simulink model "MatlabCode"  (R2017b)
settings: Solver=FixedStepDiscrete  StartTime=0.0  StopTime=inf  RelTol=1e-3
PreLoadFcn:
  | waijung.modelPreload; % Required for working with Waijung Blockset. Do not remove.
undefined symbols (not defined in the file): HSEOSC, Link, LQFP100, ST, STM32F407VG
libraries: stm32f4_io_lib x6, stm32f4_adc_lib x1, stm32f4_device_config_lib x1
(part 2 of 2)

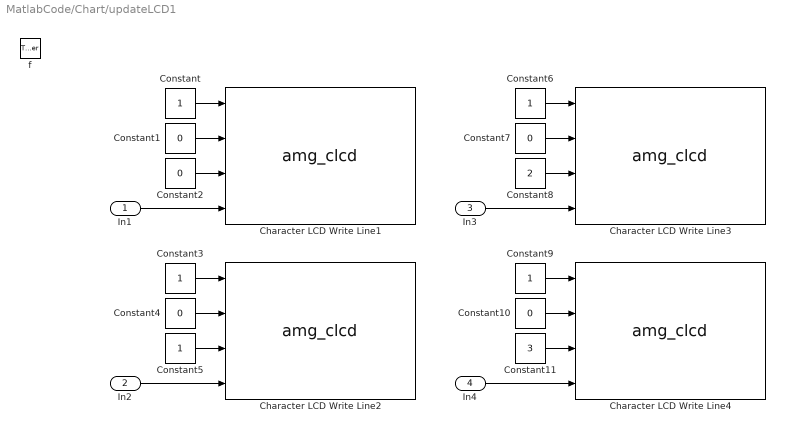
== system MatlabCode/Chart/updateLCD1 ==
  In1 : Inport  OutDataTypeStr=uint8  PortDimensions=[1 16]
  In2 : Inport  Port=2  OutDataTypeStr=uint8  PortDimensions=[1 16]
  In3 : Inport  Port=3  OutDataTypeStr=uint8  PortDimensions=[1 16]
  In4 : Inport  Port=4  OutDataTypeStr=uint8  PortDimensions=[1 16]
  f : TriggerPort  TriggerType=function-call  VariantControl=(inherit)
      settings: CopyFcn=Stateflow.SLINSF.SimulinkMan.removeBlockPreDeleteFcn  PreDeleteFcn=Stateflow.SLINSF.SimulinkMan.unsafePredeleteFcn
  Character LCD Write Line1 : S-Function  FunctionName=amg_clcd  Parameters=module,configuration,inputtypearray,outputtypearray,confstr,sampletime,sampletimestr,blockid  SFunctionDeploymentMode=off  EnableBusSupport=off  mask(amg_clcd){configuration=Transaction, module=1, model=amg CLCD Std, interface=4-bits, linecount=4, columncount=20, gpiotype=Push-pull, controlport=E, control_rs=15, control_rw=13, control_en=11, dataport=A, data0=7, data1=5, data2=3, data3=1, usestringbuffer=off, stringbuffer=<empty>, varname=, inputtypearray=[4 -1 -1 -1 -1], outputtypearray=[0], confstr=["4","4","20","PP","E","15","11","13","","A","","","","","7","5","3","1","0","","1","0","0","0","1","0","0","0","0","stm32f4"], sampletime=-1, sampletimestr=-1, blockid=ChartupdateLCD1CharacterLCDWriteLine1}
      mask prompts: model "LCD model:"; linecount "Number of lines:"; columncount "Number of columns:"; gpiotype "GPIO Output type:"; controlport "GPIO control port:"; control_rs "GPIO control pin, RS:"; control_rw "GPIO control pin, RW:"; control_en "GPIO control pin, EN:"; dataport "GPIO data D[7:4] port"; data0 "GPIO data pin, D4:"; data1 "GPIO data pin, D5:"; data2 "GPIO data pin, D6:"; data3 "GPIO data pin, D7:"; usestringbuffer "Use string buffer"; stringbuffer "String buffer"; varname "Variable name"; inputtypearray "Input type array"; outputtypearray "Output type array"; confstr "Configuration string"; sampletime "Sample time (sec)"; sampletimestr "Compiled sample time (sec) in string"
      mask help:
      | Note for cmd:
      | 1 - Clear specified LCD line display before write data to LCD.
      | Otherwise (e.g. 0) - Write data without clearing LCD Line.
      |
      | Position:
      | x = 0, First Character (from left to right)
      | y = 0, Top Line
      mask init:
      | amg_clcd_callback('init');
      mask Help: web(fullfile(waijungdocroot,'amg_clcd_write.htm'), '-browser')
      mask TypeOptions configuration: Setup | Transaction
      mask Callback configuration: amg_clcd_callback('configuration');
      mask TypeOptions module: 1 | 2 | 3 | 4
      mask TypeOptions model: amg CLCD Std
      mask TypeOptions interface: 4-bits
      mask TypeOptions gpiotype: Push-pull | Open-drain
      mask TypeOptions controlport: A | B | C | D | E | F | G | H | I
      mask TypeOptions control_rs: 0 | 1 | 2 | 3 | 4 | 5 | 6 | 7 | 8 | 9 | 10 | 11 | 12 | 13 | 14 | 15
      mask TypeOptions control_rw: 0 | 1 | 2 | 3 | 4 | 5 | 6 | 7 | 8 | 9 | 10 | 11 | 12 | 13 | 14 | 15
      mask TypeOptions control_en: 0 | 1 | 2 | 3 | 4 | 5 | 6 | 7 | 8 | 9 | 10 | 11 | 12 | 13 | 14 | 15
      mask TypeOptions dataport: A | B | C | D | E | F | G | H | I
      mask TypeOptions data0: 0 | 1 | 2 | 3 | 4 | 5 | 6 | 7 | 8 | 9 | 10 | 11 | 12 | 13 | 14 | 15
      mask TypeOptions data1: 0 | 1 | 2 | 3 | 4 | 5 | 6 | 7 | 8 | 9 | 10 | 11 | 12 | 13 | 14 | 15
      mask TypeOptions data2: 0 | 1 | 2 | 3 | 4 | 5 | 6 | 7 | 8 | 9 | 10 | 11 | 12 | 13 | 14 | 15
      mask TypeOptions data3: 0 | 1 | 2 | 3 | 4 | 5 | 6 | 7 | 8 | 9 | 10 | 11 | 12 | 13 | 14 | 15
      mask Callback usestringbuffer: amg_clcd_callback('usestringbuffer');
      mask TypeOptions stringbuffer: <empty>
      mask Callback varname: amg_clcd_callback('varname');
      mask Callback confstr: amg_clcd_callback('confstr');
      mask Callback sampletime: amg_clcd_callback('sampletime');
      mask Callback sampletimestr: amg_clcd_callback('sampletimestr');
      mask Callback blockid: amg_clcd_callback('blockid');
      mask Display: text(0.5, 0.5, 'Module: CLCD1 (Write)\nTs (sec): -1','ver','middle','hor','center');port_label('input', 1,'cmd');port_label('input', 2,'xpos');port_label('input', 3,'ypos');port_label('input', 4,'str');
  Character LCD Write Line2 : S-Function  FunctionName=amg_clcd  Parameters=module,configuration,inputtypearray,outputtypearray,confstr,sampletime,sampletimestr,blockid  SFunctionDeploymentMode=off  EnableBusSupport=off  mask(amg_clcd){configuration=Transaction, module=1, model=amg CLCD Std, interface=4-bits, linecount=4, columncount=20, gpiotype=Push-pull, controlport=E, control_rs=15, control_rw=13, control_en=11, dataport=A, data0=7, data1=5, data2=3, data3=1, usestringbuffer=off, stringbuffer=<empty>, varname=, inputtypearray=[4 -1 -1 -1 -1], outputtypearray=[0], confstr=["4","4","20","PP","E","15","11","13","","A","","","","","7","5","3","1","0","","1","0","0","0","1","0","0","0","0","stm32f4"], sampletime=-1, sampletimestr=-1, blockid=ChartupdateLCD1CharacterLCDWriteLine2}
      mask prompts: model "LCD model:"; linecount "Number of lines:"; columncount "Number of columns:"; gpiotype "GPIO Output type:"; controlport "GPIO control port:"; control_rs "GPIO control pin, RS:"; control_rw "GPIO control pin, RW:"; control_en "GPIO control pin, EN:"; dataport "GPIO data D[7:4] port"; data0 "GPIO data pin, D4:"; data1 "GPIO data pin, D5:"; data2 "GPIO data pin, D6:"; data3 "GPIO data pin, D7:"; usestringbuffer "Use string buffer"; stringbuffer "String buffer"; varname "Variable name"; inputtypearray "Input type array"; outputtypearray "Output type array"; confstr "Configuration string"; sampletime "Sample time (sec)"; sampletimestr "Compiled sample time (sec) in string"
      mask help:
      | Note for cmd:
      | 1 - Clear specified LCD line display before write data to LCD.
      | Otherwise (e.g. 0) - Write data without clearing LCD Line.
      |
      | Position:
      | x = 0, First Character (from left to right)
      | y = 0, Top Line
      mask init:
      | amg_clcd_callback('init');
      mask Help: web(fullfile(waijungdocroot,'amg_clcd_write.htm'), '-browser')
      mask TypeOptions configuration: Setup | Transaction
      mask Callback configuration: amg_clcd_callback('configuration');
      mask TypeOptions module: 1 | 2 | 3 | 4
      mask TypeOptions model: amg CLCD Std
      mask TypeOptions interface: 4-bits
      mask TypeOptions gpiotype: Push-pull | Open-drain
      mask TypeOptions controlport: A | B | C | D | E | F | G | H | I
      mask TypeOptions control_rs: 0 | 1 | 2 | 3 | 4 | 5 | 6 | 7 | 8 | 9 | 10 | 11 | 12 | 13 | 14 | 15
      mask TypeOptions control_rw: 0 | 1 | 2 | 3 | 4 | 5 | 6 | 7 | 8 | 9 | 10 | 11 | 12 | 13 | 14 | 15
      mask TypeOptions control_en: 0 | 1 | 2 | 3 | 4 | 5 | 6 | 7 | 8 | 9 | 10 | 11 | 12 | 13 | 14 | 15
      mask TypeOptions dataport: A | B | C | D | E | F | G | H | I
      mask TypeOptions data0: 0 | 1 | 2 | 3 | 4 | 5 | 6 | 7 | 8 | 9 | 10 | 11 | 12 | 13 | 14 | 15
      mask TypeOptions data1: 0 | 1 | 2 | 3 | 4 | 5 | 6 | 7 | 8 | 9 | 10 | 11 | 12 | 13 | 14 | 15
      mask TypeOptions data2: 0 | 1 | 2 | 3 | 4 | 5 | 6 | 7 | 8 | 9 | 10 | 11 | 12 | 13 | 14 | 15
      mask TypeOptions data3: 0 | 1 | 2 | 3 | 4 | 5 | 6 | 7 | 8 | 9 | 10 | 11 | 12 | 13 | 14 | 15
      mask Callback usestringbuffer: amg_clcd_callback('usestringbuffer');
      mask TypeOptions stringbuffer: <empty>
      mask Callback varname: amg_clcd_callback('varname');
      mask Callback confstr: amg_clcd_callback('confstr');
      mask Callback sampletime: amg_clcd_callback('sampletime');
      mask Callback sampletimestr: amg_clcd_callback('sampletimestr');
      mask Callback blockid: amg_clcd_callback('blockid');
      mask Display: text(0.5, 0.5, 'Module: CLCD1 (Write)\nTs (sec): -1','ver','middle','hor','center');port_label('input', 1,'cmd');port_label('input', 2,'xpos');port_label('input', 3,'ypos');port_label('input', 4,'str');
  Character LCD Write Line3 : S-Function  FunctionName=amg_clcd  Parameters=module,configuration,inputtypearray,outputtypearray,confstr,sampletime,sampletimestr,blockid  SFunctionDeploymentMode=off  EnableBusSupport=off  mask(amg_clcd){configuration=Transaction, module=1, model=amg CLCD Std, interface=4-bits, linecount=4, columncount=20, gpiotype=Push-pull, controlport=E, control_rs=15, control_rw=13, control_en=11, dataport=A, data0=7, data1=5, data2=3, data3=1, usestringbuffer=off, stringbuffer=<empty>, varname=, inputtypearray=[4 -1 -1 -1 -1], outputtypearray=[0], confstr=["4","4","20","PP","E","15","11","13","","A","","","","","7","5","3","1","0","","1","0","0","0","1","0","0","0","0","stm32f4"], sampletime=-1, sampletimestr=-1, blockid=ChartupdateLCD1CharacterLCDWriteLine3}
      mask prompts: model "LCD model:"; linecount "Number of lines:"; columncount "Number of columns:"; gpiotype "GPIO Output type:"; controlport "GPIO control port:"; control_rs "GPIO control pin, RS:"; control_rw "GPIO control pin, RW:"; control_en "GPIO control pin, EN:"; dataport "GPIO data D[7:4] port"; data0 "GPIO data pin, D4:"; data1 "GPIO data pin, D5:"; data2 "GPIO data pin, D6:"; data3 "GPIO data pin, D7:"; usestringbuffer "Use string buffer"; stringbuffer "String buffer"; varname "Variable name"; inputtypearray "Input type array"; outputtypearray "Output type array"; confstr "Configuration string"; sampletime "Sample time (sec)"; sampletimestr "Compiled sample time (sec) in string"
      mask help:
      | Note for cmd:
      | 1 - Clear specified LCD line display before write data to LCD.
      | Otherwise (e.g. 0) - Write data without clearing LCD Line.
      |
      | Position:
      | x = 0, First Character (from left to right)
      | y = 0, Top Line
      mask init:
      | amg_clcd_callback('init');
      mask Help: web(fullfile(waijungdocroot,'amg_clcd_write.htm'), '-browser')
      mask TypeOptions configuration: Setup | Transaction
      mask Callback configuration: amg_clcd_callback('configuration');
      mask TypeOptions module: 1 | 2 | 3 | 4
      mask TypeOptions model: amg CLCD Std
      mask TypeOptions interface: 4-bits
      mask TypeOptions gpiotype: Push-pull | Open-drain
      mask TypeOptions controlport: A | B | C | D | E | F | G | H | I
      mask TypeOptions control_rs: 0 | 1 | 2 | 3 | 4 | 5 | 6 | 7 | 8 | 9 | 10 | 11 | 12 | 13 | 14 | 15
      mask TypeOptions control_rw: 0 | 1 | 2 | 3 | 4 | 5 | 6 | 7 | 8 | 9 | 10 | 11 | 12 | 13 | 14 | 15
      mask TypeOptions control_en: 0 | 1 | 2 | 3 | 4 | 5 | 6 | 7 | 8 | 9 | 10 | 11 | 12 | 13 | 14 | 15
      mask TypeOptions dataport: A | B | C | D | E | F | G | H | I
      mask TypeOptions data0: 0 | 1 | 2 | 3 | 4 | 5 | 6 | 7 | 8 | 9 | 10 | 11 | 12 | 13 | 14 | 15
      mask TypeOptions data1: 0 | 1 | 2 | 3 | 4 | 5 | 6 | 7 | 8 | 9 | 10 | 11 | 12 | 13 | 14 | 15
      mask TypeOptions data2: 0 | 1 | 2 | 3 | 4 | 5 | 6 | 7 | 8 | 9 | 10 | 11 | 12 | 13 | 14 | 15
      mask TypeOptions data3: 0 | 1 | 2 | 3 | 4 | 5 | 6 | 7 | 8 | 9 | 10 | 11 | 12 | 13 | 14 | 15
      mask Callback usestringbuffer: amg_clcd_callback('usestringbuffer');
      mask TypeOptions stringbuffer: <empty>
      mask Callback varname: amg_clcd_callback('varname');
      mask Callback confstr: amg_clcd_callback('confstr');
      mask Callback sampletime: amg_clcd_callback('sampletime');
      mask Callback sampletimestr: amg_clcd_callback('sampletimestr');
      mask Callback blockid: amg_clcd_callback('blockid');
      mask Display: text(0.5, 0.5, 'Module: CLCD1 (Write)\nTs (sec): -1','ver','middle','hor','center');port_label('input', 1,'cmd');port_label('input', 2,'xpos');port_label('input', 3,'ypos');port_label('input', 4,'str');
  Character LCD Write Line4 : S-Function  FunctionName=amg_clcd  Parameters=module,configuration,inputtypearray,outputtypearray,confstr,sampletime,sampletimestr,blockid  SFunctionDeploymentMode=off  EnableBusSupport=off  mask(amg_clcd){configuration=Transaction, module=1, model=amg CLCD Std, interface=4-bits, linecount=4, columncount=20, gpiotype=Push-pull, controlport=E, control_rs=15, control_rw=13, control_en=11, dataport=A, data0=7, data1=5, data2=3, data3=1, usestringbuffer=off, stringbuffer=<empty>, varname=, inputtypearray=[4 -1 -1 -1 -1], outputtypearray=[0], confstr=["4","4","20","PP","E","15","11","13","","A","","","","","7","5","3","1","0","","1","0","0","0","1","0","0","0","0","stm32f4"], sampletime=-1, sampletimestr=-1, blockid=ChartupdateLCD1CharacterLCDWriteLine4}
      mask prompts: model "LCD model:"; linecount "Number of lines:"; columncount "Number of columns:"; gpiotype "GPIO Output type:"; controlport "GPIO control port:"; control_rs "GPIO control pin, RS:"; control_rw "GPIO control pin, RW:"; control_en "GPIO control pin, EN:"; dataport "GPIO data D[7:4] port"; data0 "GPIO data pin, D4:"; data1 "GPIO data pin, D5:"; data2 "GPIO data pin, D6:"; data3 "GPIO data pin, D7:"; usestringbuffer "Use string buffer"; stringbuffer "String buffer"; varname "Variable name"; inputtypearray "Input type array"; outputtypearray "Output type array"; confstr "Configuration string"; sampletime "Sample time (sec)"; sampletimestr "Compiled sample time (sec) in string"
      mask help:
      | Note for cmd:
      | 1 - Clear specified LCD line display before write data to LCD.
      | Otherwise (e.g. 0) - Write data without clearing LCD Line.
      |
      | Position:
      | x = 0, First Character (from left to right)
      | y = 0, Top Line
      mask init:
      | amg_clcd_callback('init');
      mask Help: web(fullfile(waijungdocroot,'amg_clcd_write.htm'), '-browser')
      mask TypeOptions configuration: Setup | Transaction
      mask Callback configuration: amg_clcd_callback('configuration');
      mask TypeOptions module: 1 | 2 | 3 | 4
      mask TypeOptions model: amg CLCD Std
      mask TypeOptions interface: 4-bits
      mask TypeOptions gpiotype: Push-pull | Open-drain
      mask TypeOptions controlport: A | B | C | D | E | F | G | H | I
      mask TypeOptions control_rs: 0 | 1 | 2 | 3 | 4 | 5 | 6 | 7 | 8 | 9 | 10 | 11 | 12 | 13 | 14 | 15
      mask TypeOptions control_rw: 0 | 1 | 2 | 3 | 4 | 5 | 6 | 7 | 8 | 9 | 10 | 11 | 12 | 13 | 14 | 15
      mask TypeOptions control_en: 0 | 1 | 2 | 3 | 4 | 5 | 6 | 7 | 8 | 9 | 10 | 11 | 12 | 13 | 14 | 15
      mask TypeOptions dataport: A | B | C | D | E | F | G | H | I
      mask TypeOptions data0: 0 | 1 | 2 | 3 | 4 | 5 | 6 | 7 | 8 | 9 | 10 | 11 | 12 | 13 | 14 | 15
      mask TypeOptions data1: 0 | 1 | 2 | 3 | 4 | 5 | 6 | 7 | 8 | 9 | 10 | 11 | 12 | 13 | 14 | 15
      mask TypeOptions data2: 0 | 1 | 2 | 3 | 4 | 5 | 6 | 7 | 8 | 9 | 10 | 11 | 12 | 13 | 14 | 15
      mask TypeOptions data3: 0 | 1 | 2 | 3 | 4 | 5 | 6 | 7 | 8 | 9 | 10 | 11 | 12 | 13 | 14 | 15
      mask Callback usestringbuffer: amg_clcd_callback('usestringbuffer');
      mask TypeOptions stringbuffer: <empty>
      mask Callback varname: amg_clcd_callback('varname');
      mask Callback confstr: amg_clcd_callback('confstr');
      mask Callback sampletime: amg_clcd_callback('sampletime');
      mask Callback sampletimestr: amg_clcd_callback('sampletimestr');
      mask Callback blockid: amg_clcd_callback('blockid');
      mask Display: text(0.5, 0.5, 'Module: CLCD1 (Write)\nTs (sec): -1','ver','middle','hor','center');port_label('input', 1,'cmd');port_label('input', 2,'xpos');port_label('input', 3,'ypos');port_label('input', 4,'str');
  Constant{,3,5..6,9} (5 alike) : Constant
  Constant{1..2,4,7,10} (5 alike) : Constant  Value=0
  Constant11 : Constant  Value=3
  Constant8 : Constant  Value=2
  wires:
  In1/1 -> Character LCD Write Line1/4
  Constant/1 -> Character LCD Write Line1/1
  Constant1/1 -> Character LCD Write Line1/2
  Constant2/1 -> Character LCD Write Line1/3
  In2/1 -> Character LCD Write Line2/4
  Constant3/1 -> Character LCD Write Line2/1
  Constant4/1 -> Character LCD Write Line2/2
  Constant5/1 -> Character LCD Write Line2/3
  In3/1 -> Character LCD Write Line3/4
  Constant6/1 -> Character LCD Write Line3/1
  Constant7/1 -> Character LCD Write Line3/2
  Constant8/1 -> Character LCD Write Line3/3
  In4/1 -> Character LCD Write Line4/4
  Constant9/1 -> Character LCD Write Line4/1
  Constant10/1 -> Character LCD Write Line4/2
  Constant11/1 -> Character LCD Write Line4/3

== stateflow chart MatlabCode/Chart ==
  state Initialization
  state NormalOperation
    state CheckKeyPress [parallel]
      settings: executionOrder=2
      state NoKeyPressed
        en: data = 0;
      state UpKeyPressed
        en: data = 1;
        state Short
        state Long
        state Break
        (default) -> NormalOperation.CheckKeyPress.UpKeyPressed.Short : {UP_KEY_PRESSED;}
        NormalOperation.CheckKeyPress.UpKeyPressed.Short -> NormalOperation.CheckKeyPress.UpKeyPressed.Long : after(1,sec)
        NormalOperation.CheckKeyPress.UpKeyPressed.Long -> NormalOperation.CheckKeyPress.UpKeyPressed.Break
      state DownKeyPressed
        en: data = 1;
        state Short
        state Long
        state Break
        (default) -> NormalOperation.CheckKeyPress.DownKeyPressed.Short : {DOWN_KEY_PRESSED;}
        NormalOperation.CheckKeyPress.DownKeyPressed.Short -> NormalOperation.CheckKeyPress.DownKeyPressed.Long : after(1,sec)
        NormalOperation.CheckKeyPress.DownKeyPressed.Long -> NormalOperation.CheckKeyPress.DownKeyPressed.Break
      state OkKeyPressed
        en: data = 1;
        state Short
        (default) -> NormalOperation.CheckKeyPress.OkKeyPressed.Short : {OK_KEY_PRESSED;}
      (default) -> NoKeyPressed
      NoKeyPressed -> UpKeyPressed [order 1] : [up_key == 1]
      UpKeyPressed -> NoKeyPressed : [up_key == 0]
      NoKeyPressed -> DownKeyPressed [order 2] : [down_key == 1]
      DownKeyPressed -> NoKeyPressed : [down_key == 0]
      NoKeyPressed -> OkKeyPressed [order 3] : [ok_key == 1]
      OkKeyPressed -> NoKeyPressed : [ok_key == 0]
    state MenuDisplay [parallel]
      settings: executionOrder=1
      state Screen1
        en: lcd_line1 = setLcdLine1(1);
        en: lcd_line2 = setLcdLine2(1);
        en: lcd_line3 = setLcdLine3(1);
        en: lcd_line4 = setLcdLine4(1);
        en: updateLCD1(lcd_line1,lcd_line2,lcd_line3,lcd_line4);
      state Screen2
        en: lcd_line1 = setLcdLine1(2);
        en: lcd_line2 = setLcdLine2(2);
        en: lcd_line3 = setLcdLine3(2);
        en: lcd_line4 = setLcdLine4(2);
        en: updateLCD1(lcd_line1,lcd_line2,lcd_line3,lcd_line4);
      state Screen4
        en: lcd_line1 = setLcdLine1(4);
        en: TotalDate();
        en: StartDate();
        en: lcd_line4 = setLcdLine4(0);
        en: updateLCD1(lcd_line1,lcd_line2,lcd_line3,lcd_line4);
      state Screen21
        en: lcd_line1 = setLcdLine1(21);
        en: lcd_line2 = setLcdLine2(21);
        en: lcd_line3 = setLcdLine3(2);
        en: lcd_line4 = setLcdLine4(2);
        en: updateLCD1(lcd_line1,lcd_line2,lcd_line3,lcd_line4);
      state Screen5
        en: lcd_line1 = setLcdLine1(5);
        en: lcd_line2 = setLcdLine2(5);
        en: SetTimeHH();
        en: SetTimeMM();
        en: updateLCD1(lcd_line1,lcd_line2,lcd_line3,lcd_line4);
      state Screen51
        en: MoisSlide();
        en: FerASec();
        en: FerBSec();
        en: lcd_line4 = setLcdLine4(0);
        en: updateLCD1(lcd_line1,lcd_line2,lcd_line3,lcd_line4);
      state Screen22
        en: lcd_line1 = setLcdLine1(21);
        en: lcd_line2 = setLcdLine2(2);
        en: lcd_line3 = setLcdLine3(21);
        en: lcd_line4 = setLcdLine4(2);
        en: updateLCD1(lcd_line1,lcd_line2,lcd_line3,lcd_line4);
      state Screen6
        en: lcd_line1 = setLcdLine1(6);
        en: SetMois();
        en: FerAStatus();
        en: FerBStatus();
        en: updateLCD1(lcd_line1,lcd_line2,lcd_line3,lcd_line4);
      state Screen61
        en: ValveStatus();
        en: lcd_line2 = setLcdLine2(0);
        en: lcd_line3 = setLcdLine3(0);
        en: lcd_line4 = setLcdLine4(0);
        en: updateLCD1(lcd_line1,lcd_line2,lcd_line3,lcd_line4);
      state Screen23
        en: lcd_line1 = setLcdLine1(21);
        en: lcd_line2 = setLcdLine2(2);
        en: lcd_line3 = setLcdLine3(2);
        en: lcd_line4 = setLcdLine4(21);
        en: updateLCD1(lcd_line1,lcd_line2,lcd_line3,lcd_line4);
      state Screen7
        en: lcd_line1 = setLcdLine1(7);
        en: FerAControl();
        en: FerBControl();
        en: ValveControl();
        en: updateLCD1(lcd_line1,lcd_line2,lcd_line3,lcd_line4);
      state Screen3
        en: lcd_line1 = setLcdLine1(3);
        en: lcd_line2 = setLcdLine2(3);
        en: lcd_line3 = setLcdLine3(0);
        en: lcd_line4 = setLcdLine4(3);
        en: updateLCD1(lcd_line1,lcd_line2,lcd_line3,lcd_line4);
      state Screen8
        en: lcd_line1 = setLcdLine1(8);
        en: RSetTimeHH();
        en: RSetTimeMM();
        en: RSetTimeSS();
        en: updateLCD1(lcd_line1,lcd_line2,lcd_line3,lcd_line4);
      state Screen81
        en: RSetDay();
        en: RSetMonth();
        en: RSetYear();
        en: lcd_line4 = setLcdLine4(0);
        en: updateLCD1(lcd_line1,lcd_line2,lcd_line3,lcd_line4);
      state Screen31
        en: lcd_line1 = setLcdLine1(31);
        en: lcd_line2 = setLcdLine2(31);
        en: lcd_line3 = setLcdLine3(0);
        en: lcd_line4 = setLcdLine4(3);
        en: updateLCD1(lcd_line1,lcd_line2,lcd_line3,lcd_line4);
      state Screen32
        en: lcd_line1 = setLcdLine1(31);
        en: lcd_line2 = setLcdLine2(3);
        en: lcd_line3 = setLcdLine3(0);
        en: lcd_line4 = setLcdLine4(31);
        en: updateLCD1(lcd_line1,lcd_line2,lcd_line3,lcd_line4);
      Screen4 -> Screen4 [order 2] : after(0.5,sec)
      (default) -> Screen1
      Screen2 -> Screen4 [order 2] : OK_KEY_PRESSED
      Screen2 -> Screen1 [order 3] : [in(CheckKeyPress.UpKeyPressed.Long)]
      Screen4 -> Screen2 [order 1] : [in(CheckKeyPress.UpKeyPressed.Long)]
      Screen1 -> Screen2 : OK_KEY_PRESSED
      Screen2 -> Screen21 [order 1] : DOWN_KEY_PRESSED
      Screen21 -> Screen2 [order 1] : UP_KEY_PRESSED
      Screen23 -> Screen1 [order 3] : [in(CheckKeyPress.DownKeyPressed.Long)]
      Screen5 -> Screen5 [order 3] : after(0.5,sec)
      Screen51 -> Screen51 [order 3] : after(0.5,sec)
      Screen21 -> Screen5 [order 3] : OK_KEY_PRESSED
      Screen51 -> Screen5 [order 1] : UP_KEY_PRESSED
      Screen5 -> Screen21 [order 1] : [in(CheckKeyPress.UpKeyPressed.Long)]
      Screen5 -> Screen51 [order 2] : DOWN_KEY_PRESSED
      Screen21 -> Screen22 [order 2] : DOWN_KEY_PRESSED
      Screen22 -> Screen21 [order 1] : UP_KEY_PRESSED
      Screen51 -> Screen21 [order 2] : [in(CheckKeyPress.DownKeyPressed.Long)]
      Screen6 -> Screen6 [order 3] : after(0.5,sec)
      Screen61 -> Screen61 [order 3] : after(0.5,sec)
      Screen22 -> Screen6 [order 3] : OK_KEY_PRESSED
      Screen61 -> Screen6 [order 1] : UP_KEY_PRESSED
      Screen6 -> Screen22 [order 1] : [in(CheckKeyPress.UpKeyPressed.Long)]
      Screen6 -> Screen61 [order 2] : DOWN_KEY_PRESSED
      Screen22 -> Screen23 [order 2] : DOWN_KEY_PRESSED
      Screen61 -> Screen22 [order 2] : [in(CheckKeyPress.DownKeyPressed.Long)]
      Screen23 -> Screen22 [order 1] : UP_KEY_PRESSED
      Screen32 -> Screen23 [order 2] : OK_KEY_PRESSED
      Screen7 -> Screen3 [order 3] : DOWN_KEY_PRESSED
      Screen23 -> Screen3 [order 2] : OK_KEY_PRESSED
      Screen7 -> Screen7 [order 2] : after(0.5,sec)
      Screen3 -> Screen7 [order 2] : OK_KEY_PRESSED
      Screen7 -> Screen3 [order 1] : [in(CheckKeyPress.UpKeyPressed.Long)]
      Screen3 -> Screen31 [order 1] : DOWN_KEY_PRESSED
      Screen31 -> Screen3 [order 1] : UP_KEY_PRESSED
      Screen8 -> Screen8 [order 3] : after(0.5,sec)
      Screen81 -> Screen81 [order 2] : after(0.5,sec)
      Screen31 -> Screen8 [order 3] : OK_KEY_PRESSED
      Screen81 -> Screen8 [order 1] : UP_KEY_PRESSED
      Screen8 -> Screen81 [order 2] : DOWN_KEY_PRESSED
      Screen8 -> Screen31 [order 1] : [in(CheckKeyPress.UpKeyPressed.Long)]
      Screen81 -> Screen31 [order 3] : [in(CheckKeyPress.DownKeyPressed.Long)]
      Screen31 -> Screen32 [order 2] : DOWN_KEY_PRESSED
      Screen32 -> Screen31 [order 1] : UP_KEY_PRESSED
  state updateLCD1(In1,In2,In3,In4) [function]
  (default) -> Initialization
  Initialization -> NormalOperation
  data: option function_input double; outstr function_output uint8 size=[1 16]; option function_input double; outstr function_output uint8 size=[1 16]; option function_input double; outstr function_output uint8 size=[1 16]; option function_input double; outstr function_output uint8 size=[1 16]; In1 function_input uint8 size=[1 16]; In2 function_input uint8 size=[1 16]; In3 function_input uint8 size=[1 16]; In4 function_input uint8 size=[1 16]; ok_key input; up_key input; down_key input; data output double =0; lcd_line1 local uint8 size=[1 16]; lcd_line2 local uint8 size=[1 16]; lcd_line3 local uint8 size=[1 16]; lcd_line4 local uint8 size=[1 16]; Mois input double; button_V31 input; button_V32 input; button_V33 input; Hour input; Minute input; Total input; Start input; Mois2 input double; FerA input double; FerB input double; FerAS input; FerBS input; ValveS input; Hour2 input; Minute2 input; Second2 input; Day input; Year input
  events: triger input RISING_EDGE_EVENT; UP_KEY_PRESSED local FUNCTION_CALL_EVENT; OK_KEY_PRESSED local FUNCTION_CALL_EVENT; DOWN_KEY_PRESSED local FUNCTION_CALL_EVENT
  function outstr = setLcdLine1(option):
    | function outstr = setLcdLine1(option)
    | 
    | switch option
    |     case 0             %0123456789ABCDEF
    |         outstr = uint8('                ');
    |     case 1  
    |         outstr = uint8('  SMF-AUTOMATIC ');
    |     case 2 
    |         outstr = uint8('>MAIN SCREEN    ');
    |     case 21 
    |         outstr = uint8(' MAIN SCREEN    ');
    |     case 3 
    |         outstr = uint8('>MANUAL SCREEN  ');
    |     case 31 
    |         outstr = uint8(' MANUAL SCREEN  ');
    |     case 4 
    |         outstr = uint8('   ** MAIN **   ');
    |     case 5 
    |         outstr = uint8('  ** CONFIG **  ');
    |     case 6 
    |         outstr = uint8('  **MONITOR**   ');
    |     case 61
    |         outstr = uint8('SoleNoidValve:  ');
    |     case 7 
    |         outstr = uint8('   **MANUAL**   ');
    |     case 8 
    |         outstr = uint8('  **SET-TIME**  ');
    |     case 81 
    |         outstr = uint8('SET-DAY:      HH');
    |     
    |     otherwise
    |         outstr = uint8('                ');
    | end
  function outstr = setLcdLine2(option):
    | function outstr = setLcdLine2(option)
    | 
    | switch option
    |     case 0             %0123456789ABCDEF
    |         outstr = uint8('                ');
    |     case 1  
    |         outstr = uint8(' WATERING SYSTEM');
    |     case 2 
    |         outstr = uint8(' CONFIG SCREEN  ');
    |     case 21 
    |         outstr = uint8('>CONFIG SCREEN  ');
    |     case 3
    |         outstr = uint8(' SET-TIME SCREEN');
    |     case 31
    |         outstr = uint8('>SET-TIME SCREEN');
    |     case 4 
    |         outstr = uint8('TOTAL DATE:     ');
    |     case 5 
    |         outstr = uint8('Easy            ');
    |     case 7 
    |         outstr = uint8('FerA(Status):   ');
    |     case 8 
    |         outstr = uint8('SET-TIME:     HH');
    |     case 81 
    |         outstr = uint8('SET-DAY:      MM');
    |  
    |     
    |     otherwise
    |         outstr = uint8('                ');
    | end
  function TotalDate:
    | function TotalDate
    | coder.ceval('sprintf',coder.ref(lcd_line2), ['TotalDate:     %.0f '],Total);
  function ValveControl:
    | function ValveControl
    |    
    |        switch button_V33
    |            case 0
    |            coder.ceval('sprintf',coder.ref(lcd_line4), ['Valve :OFF'],button_V33);
    |            case 1
    |            coder.ceval('sprintf',coder.ref(lcd_line4), ['Valve        :ON '],button_V33);
    |                                                    
    |        end
  function SetTimeHH:
    | function SetTimeHH
    | coder.ceval('sprintf',coder.ref(lcd_line3), ['Time:      %02.0f HH'],Hour);
  function SetTimeMM:
    | function SetTimeMM
    | coder.ceval('sprintf',coder.ref(lcd_line4), ['           %02.0f MM'],Minute);
  function SetMois:
    | function SetMois
    | coder.ceval('sprintf',coder.ref(lcd_line2), ('MOISTURE: %04.1f %% '),Mois);
  function FerAControl:
    | function FerAControl
    |    
    |        switch button_V31
    |            case 0
    |            coder.ceval('sprintf',coder.ref(lcd_line2), ['FerA(Status):OFF'],button_V31);
    |            case 1
    |            coder.ceval('sprintf',coder.ref(lcd_line2), ['FerA(Status):ON '],button_V31);
    |                                                    
    |        end
  function FerBControl:
    | function FerBControl
    |    
    |        switch button_V32
    |            case 0
    |            coder.ceval('sprintf',coder.ref(lcd_line3), ['FerB(Status):OFF'],button_V32);
    |            case 1
    |            coder.ceval('sprintf',coder.ref(lcd_line3), ['FerB(Status):ON '],button_V32);
    |                                                    
    |        end
  function MoisSlide:
    | function MoisSlide
    | coder.ceval('sprintf',coder.ref(lcd_line1), ('MOISTURE:  %02.0f %% '),Mois2);
  function FerASec:
    | function FerASec
    | coder.ceval('sprintf',coder.ref(lcd_line2), ('FerA(s)=   %.0f sec'),FerA);
  function FerBSec:
    | function FerBSec
    | coder.ceval('sprintf',coder.ref(lcd_line3), ('FerB(s)=   %.0f sec'),FerB);
  function FerAStatus:
    | function FerAStatus
    |   switch FerAS
    |            case 0
    |            coder.ceval('sprintf',coder.ref(lcd_line3), ['FerA(Status):OFF'],FerAS);
    |            case 1
    |            coder.ceval('sprintf',coder.ref(lcd_line3), ['FerA(Status):ON '],FerAS);
    |                                                    
    |   end
  function FerBStatus:
    | function FerBStatus
    |   switch FerBS
    |            case 0
    |            coder.ceval('sprintf',coder.ref(lcd_line4), ['FerA(Status):OFF'],FerBS);
    |            case 1
    |            coder.ceval('sprintf',coder.ref(lcd_line4), ['FerA(Status):ON '],FerBS);
    |                                                    
    |   end
  function ValveStatus:
    | function ValveStatus
    |   switch ValveS
    |            case 0
    |            coder.ceval('sprintf',coder.ref(lcd_line1), ['The Valve is OFF'],ValveS);
    |            case 1
    |            coder.ceval('sprintf',coder.ref(lcd_line1), ['The Valve is ON '],ValveS);
    |                                                    
    |   end
  function StartDate:
    | function StartDate
    | coder.ceval('sprintf',coder.ref(lcd_line3), ['StartDate:     %.0f '],Start);
  function RSetTimeHH:
    | function RSetTimeHH
    | coder.ceval('sprintf',coder.ref(lcd_line2), ['Set-Time:  %02.0f HH'],Hour2);
  function RSetTimeMM:
    | function RSetTimeMM
    | coder.ceval('sprintf',coder.ref(lcd_line3), ['           %02.0f MM'],Minute2);
  function RSetTimeSS:
    | function RSetTimeSS
    | coder.ceval('sprintf',coder.ref(lcd_line4), ['           %02.0f SS'],Second2);
  function RSetDay:
    | function RSetDay
    | coder.ceval('sprintf',coder.ref(lcd_line1), ['Set-Date:  %02.0f  D'],Day);
  function RSetMonth:
    | function RSetMonth
    | coder.ceval('sprintf',coder.ref(lcd_line2), ['           %02.0f  M'],Month);
  function RSetYear:
    | function RSetYear
    | coder.ceval('sprintf',coder.ref(lcd_line3), ['           %02.0f  Y'],Year);
  function outstr = setLcdLine3(option):
    | function outstr = setLcdLine3(option)
    | 
    | switch option
    |     case 0             %0123456789ABCDEF
    |         outstr = uint8('                ');
    |     case 1  
    |         outstr = uint8(' Voramet&Tanagon');
    |     case 2 
    |         outstr = uint8(' MONITOR SCREEN ');
    |     case 21 
    |         outstr = uint8('>MONITOR SCREEN ');
    |     case 4 
    |         outstr = uint8('START DATE:     ');
    |     case 7 
    |         outstr = uint8('FerB(Status):   ');
    |     case 8 
    |         outstr = uint8('SET-TIME:     MM');
    |     case 81 
    |         outstr = uint8('SET-DAY:      SS');
    | 
    |     otherwise
    |         outstr = uint8('                ');
    | end
  function outstr = setLcdLine4(option):
    | function outstr = setLcdLine4(option)
    | 
    | switch option
    |     case 0             %0123456789ABCDEF
    |         outstr = uint8('                ');
    |     case 1  
    |         outstr = uint8('  EE3705(641)   ');
    |     case 2 
    |         outstr = uint8(' MORE SCREEN    ');
    |     case 21 
    |         outstr = uint8('>MORE SCREEN    ');
    |     case 3 
    |         outstr = uint8(' GO BACK        ');
    |     case 31 
    |         outstr = uint8('>GO BACK        ');
    |     case 61 
    |         outstr = uint8('FerB(Status):   ');
    |     case 7 
    |         outstr = uint8('SoleNoidValve:  ');
    |     case 8 
    |         outstr = uint8('SET-TIME:     SS');
    | 
    | 
    |     otherwise
    |         outstr = uint8('                ');
    | end
